simulink subsystem "PieroModelo"  (R2023b)
settings: Solver=VariableStepAuto  StartTime=0.0  StopTime=10.0  RelTol=1e-3
settings Model: Creator=Usuario_UMA  LastModifiedBy=alumnos

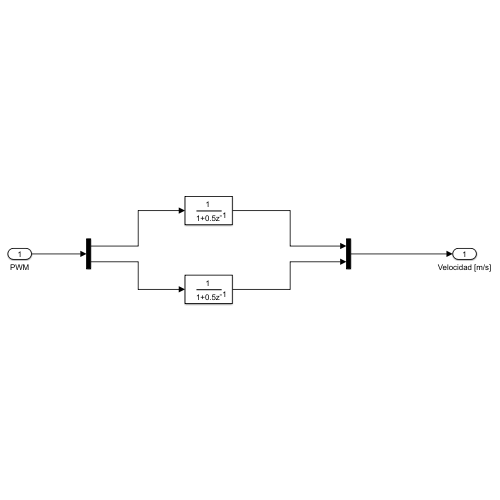
[thumbnail: Simulink's stored preview of the top-level diagram]
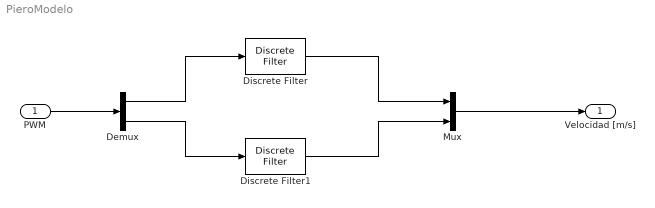
== system PieroModelo ==
  PWM : Inport
  Demux : Demux  Outputs=2
  Discrete Filter : DiscreteFilter
  Discrete Filter1 : DiscreteFilter
  Mux : Mux  Inputs=2
  Velocidad [m/s] : Outport
  wires:
  PWM/1 -> Demux/1
  Demux/1 -> Discrete Filter/1
  Discrete Filter/1 -> Mux/1
  Demux/2 -> Discrete Filter1/1
  Discrete Filter1/1 -> Mux/2
  Mux/1 -> Velocidad [m/s]/1
